simulink model "Ball_Drop_final"  (R2019b)
settings: Solver=VariableStepAuto  StartTime=0.0  StopTime=40  FixedStep=20/2160  MaxStep=0.01  RelTol=1e-3
values from neighbouring files (symbols this model uses):
  air_dens = 0    [Ball_Drop_Runner.m]
  ball_dia = 0.067    [Ball_Drop_Runner.m]
  coef_rest = 0.75    [Ball_Drop_Runner.m]
  drag_coef = 0.53    [Ball_Drop_Runner.m]
  gravity = evalin('base', 'gravity')    [Ball_Drop_Runner.m]
  init_height = 2.54    [Ball_Drop_Runner.m]
  mass = evalin('base', 'mass')    [Ball_Drop_Runner.m]
  stop_en = true    [Ball_Drop_Runner.m]
libraries: simulink x1
settings Model: Creator=qnb15169  LastModifiedBy=slam
settings SolverCC: ZeroCrossControl=EnableAll  ZeroCrossAlgorithm=Adaptive
settings DataIOCC: ReturnWorkspaceOutputs=off
settings DebuggingCC: ArithmeticOperatorsInVariantConditions=warning
settings SFSimCC: SimUseLocalCustomCode=off  CustomCodeUndefinedFunction=UseInterfaceOnly
settings RTWCC: RTWUseLocalCustomCode=off

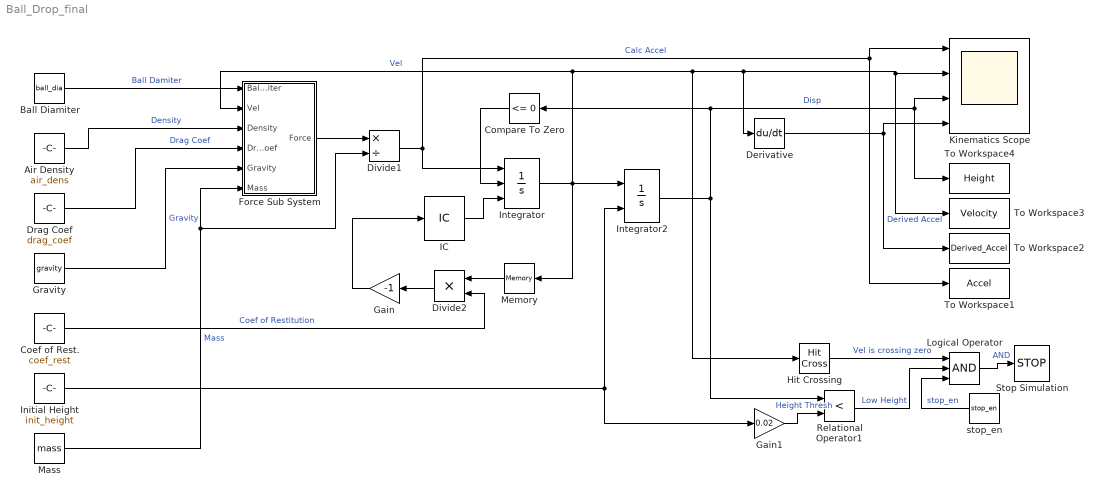
== system Ball_Drop_final ==
  "Air Density " : Constant  Value=air_dens
  Ball Diamiter : Constant  Value=ball_dia
  Coef of Rest. : Constant  Value=coef_rest
  Compare To Zero : simulink/Logic and Bit Operations/Compare To Zero  relop=<=  OutDataTypeStr=boolean
  Derivative : Derivative
  Divide1 : Product  Inputs=*/
  Divide2 : Product  Inputs=**
  Drag Coef : Constant  Value=drag_coef
  Force Sub System : Subsystem
  Gain : Gain  Gain=-1
  Gain1 : Gain  Gain=0.02
  "Gravity " : Constant  Value=gravity
  Hit Crossing : HitCross  HitCrossingDirection=falling
  IC : InitialCondition  Value=0
  Initial Height : Constant  Value=init_height
  Integrator : Integrator  ExternalReset=rising  InitialConditionSource=external
  Integrator2 : Integrator  InitialConditionSource=external  LimitOutput=on  LowerSaturationLimit=0
  Kinematics Scope : Scope  NumInputPorts=4
  Logical Operator : Logic  Inputs=3  IconShape=distinctive  AllPortsSameDT=off  OutDataTypeStr=boolean
  Mass : Constant  Value=mass
  Memory : Memory
  Relational Operator1 : RelationalOperator  Operator=<  OutDataTypeStr=boolean  RndMeth=Simplest
  Stop Simulation : Stop
  To Workspace1 : ToWorkspace  VariableName=Accel  SaveFormat=Structure With Time  SampleTime=-1
  To Workspace2 : ToWorkspace  VariableName=Derived_Accel  SaveFormat=Structure With Time  SampleTime=-1
  To Workspace3 : ToWorkspace  VariableName=Velocity  SaveFormat=Structure With Time  SampleTime=-1
  To Workspace4 : ToWorkspace  VariableName=Height  SaveFormat=Structure With Time  SampleTime=-1
  stop_en : Constant  Value=stop_en
  wires:
  Integrator/1 -> Hit Crossing/1, Derivative/1, To Workspace3/1, Kinematics Scope/2, Force Sub System/2(Vel), Integrator2/1, Memory/1  "Vel"
  Gain/1 -> IC/1
  IC/1 -> Integrator/3
  Compare To Zero/1 -> Integrator/2
  Integrator2/1 -> Relational Operator1/1, To Workspace4/1, Kinematics Scope/3, Compare To Zero/1  "Disp"
  Initial Height/1 -> Gain1/1, Integrator2/2
  Mass/1 -> Divide1/2, Force Sub System/6(Mass)  "Mass"
  "Gravity "/1 -> Force Sub System/5(Gravity)  "Gravity"
  Divide1/1 -> To Workspace1/1, Kinematics Scope/1, Integrator/1  "Calc Accel"
  Ball Diamiter/1 -> Force Sub System/1(Ball Damiter)  "Ball Damiter"
  "Air Density "/1 -> Force Sub System/3(Density)  "Density"
  Drag Coef/1 -> Force Sub System/4(Drag Coef)  "Drag Coef"
  Force Sub System/1(Force) -> Divide1/1
  Derivative/1 -> To Workspace2/1, Kinematics Scope/4  "Derived Accel"
  Divide2/1 -> Gain/1
  Memory/1 -> Divide2/1
  Coef of Rest./1 -> Divide2/2  "Coef of Restitution"
  Gain1/1 -> Relational Operator1/2  "Height Thresh"
  Logical Operator/1 -> Stop Simulation/1  "AND"
  Hit Crossing/1 -> Logical Operator/1  "Vel is crossing zero"
  Relational Operator1/1 -> Logical Operator/2  "Low Height"
  stop_en/1 -> Logical Operator/3  "stop_en"

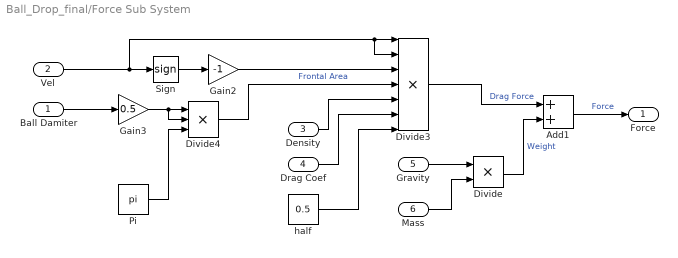
== system Ball_Drop_final/Force Sub System ==
  Ball Damiter : Inport
  Vel : Inport  Port=2
  Density : Inport  Port=3
  Drag Coef : Inport  Port=4
  Gravity : Inport  Port=5
  Mass : Inport  Port=6
  Add1 : Sum
  Divide : Product  Inputs=**
  Divide3 : Product  Inputs=*******
  Divide4 : Product  Inputs=***
  Gain2 : Gain  Gain=-1
  Gain3 : Gain  Gain=0.5
  Pi : Constant  Value=pi
  Sign : Signum
  half : Constant  Value=0.5
  Force : Outport  VectorParamsAs1DForOutWhenUnconnected=off
  wires:
  Mass/1 -> Divide/2
  Divide3/1 -> Add1/1  "Drag Force"
  Divide/1 -> Add1/2  "Weight"
  Gravity/1 -> Divide/1
  Add1/1 -> Force/1  "Force"
  half/1 -> Divide3/7
  Gain2/1 -> Divide3/3
  Density/1 -> Divide3/5
  Drag Coef/1 -> Divide3/6
  Sign/1 -> Gain2/1
  Vel/1 -> Divide3/2, Divide3/1, Sign/1
  Pi/1 -> Divide4/3
  Divide4/1 -> Divide3/4  "Frontal Area"
  Ball Damiter/1 -> Gain3/1
  Gain3/1 -> Divide4/2, Divide4/1
